simulink model "test_sim_non_linear_control_ver1"  (R2023a)
settings: Solver=FixedStepAuto  StartTime=0.0  StopTime=10.0  FixedStep=0.01  RelTol=1e-3
values from neighbouring files (symbols this model uses):
  e_init = y_init(2) - r_init(1)    [model_main_v10.m]
  K = Ke(:, 1:lenA)    [model_main_v10.m]
  KI = Ke(1, lenA+1:end)    [model_main_v10.m]
  x_init = [0 ... (first row only)    [model_main_v10.m]
libraries: simulink x2
settings Model: Creator=valer  LastModifiedBy=valer

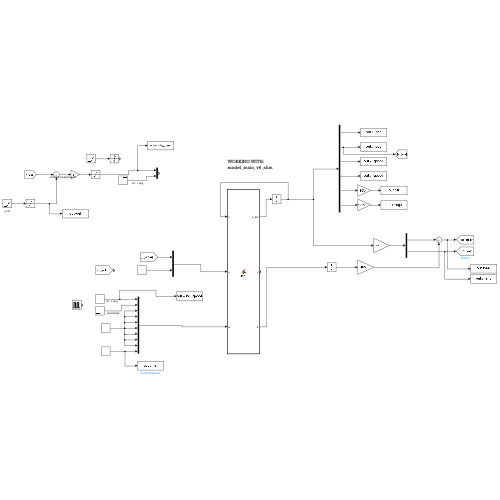
[thumbnail: Simulink's stored preview of the top-level diagram]
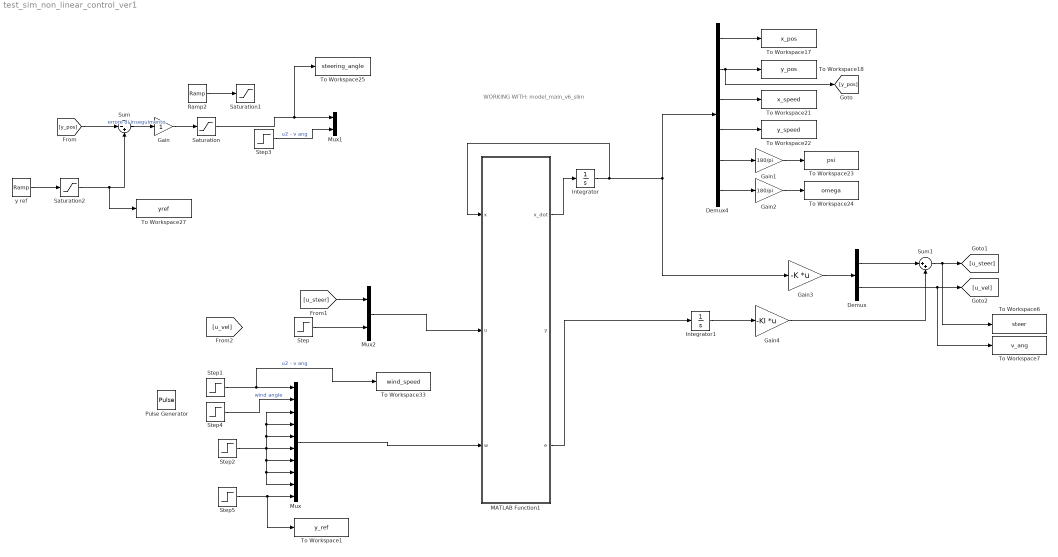
== system test_sim_non_linear_control_ver1 ==
  note: WORKING WITH:
      | model_main_v6_slim
  Demux : Demux  Outputs=2
  Demux4 : Demux  Outputs=6
  Gain : Gain
  Gain1 : Gain  Gain=180/pi
  Gain2 : Gain  Gain=180/pi
  Gain3 : Gain  Gain=-K  Multiplication=Matrix(K*u)
  Gain4 : Gain  Gain=-KI  Multiplication=Matrix(K*u)
  Integrator : Integrator  InitialCondition=x_init
  Integrator1 : Integrator  InitialCondition=e_init
  MATLAB Function1 : MATLAB Function  TreatAsAtomicUnit=on
  Mux : Mux  Inputs=10
  Mux1 : Mux  Inputs=2
  Mux2 : Mux  Inputs=2
  Pulse Generator : DiscretePulseGenerator  PulseType=Time based  Amplitude=0  Period=20  PulseWidth=50  PhaseDelay=1
  Ramp2 : simulink/Sources/Ramp  slope=0  start=1  InitialOutput=0
  Saturation : Saturate  UpperLimit=pi/4  LowerLimit=-pi/4
  Saturation1 : Saturate  UpperLimit=pi/36  LowerLimit=-pi/36
  Saturation2 : Saturate  UpperLimit=2.5  LowerLimit=-2.5
  Step : Step  Time=0  After=200  SampleTime=0
  Step1 : Step  After=0  SampleTime=0
  Step2 : Step  Time=0  Before=1  After=0  SampleTime=0
  Step3 : Step  Time=0  After=100  SampleTime=0
  Step4 : Step  After=0  SampleTime=0
  Step5 : Step  Time=0  Before=1  After=0  SampleTime=0
  Sum : Sum  Inputs=|-+
  Sum1 : Sum  Inputs=|++
  To Workspace1 : ToWorkspace  VariableName=y_ref  SaveFormat=Timeseries  SampleTime=-1
  To Workspace17 : ToWorkspace  VariableName=x_pos  SaveFormat=Timeseries  SampleTime=-1
  To Workspace18 : ToWorkspace  VariableName=y_pos  SaveFormat=Timeseries  SampleTime=-1
  To Workspace21 : ToWorkspace  VariableName=x_speed  SaveFormat=Timeseries  SampleTime=-1
  To Workspace22 : ToWorkspace  VariableName=y_speed  SaveFormat=Timeseries  SampleTime=-1
  To Workspace23 : ToWorkspace  VariableName=psi  SaveFormat=Timeseries  SampleTime=-1
  To Workspace24 : ToWorkspace  VariableName=omega  SaveFormat=Timeseries  SampleTime=-1
  To Workspace25 : ToWorkspace  VariableName=steering_angle  SaveFormat=Timeseries  SampleTime=-1
  To Workspace27 : ToWorkspace  VariableName=yref  SaveFormat=Timeseries  SampleTime=-1
  To Workspace33 : ToWorkspace  VariableName=wind_speed  SaveFormat=Timeseries  SampleTime=-1
  To Workspace6 : ToWorkspace  VariableName=steer  SaveFormat=Timeseries  SampleTime=-1
  To Workspace7 : ToWorkspace  VariableName=v_ang  SaveFormat=Timeseries  SampleTime=-1
  y ref : simulink/Sources/Ramp  slope=0  start=1  InitialOutput=0
  wires:
  Mux/1 -> MATLAB Function1/3(w)
  MATLAB Function1/1(x_dot) -> Integrator/1
  Integrator/1 -> MATLAB Function1/1(x), Gain3/1, Demux4/1
  Demux4/3 -> To Workspace21/1
  Demux4/1 -> To Workspace17/1
  Demux4/2 -> To Workspace18/1, [y_pos]
  Demux4/4 -> To Workspace22/1
  Step3/1 -> Mux1/2  "u2 - v ang"
  Step2/1 -> Mux/5, Mux/4, Mux/3, Mux/7, Mux/8, Mux/9, Mux/6
  Step4/1 -> Mux/2  "wind angle"
  [y_pos] -> Sum/1
  Sum/1 -> Gain/1  "errore di inseguimento"
  Gain/1 -> Saturation/1
  y ref/1 -> Saturation2/1
  Saturation2/1 -> To Workspace27/1, Sum/2
  Demux4/5 -> Gain1/1
  Gain2/1 -> To Workspace24/1
  Gain1/1 -> To Workspace23/1
  Demux4/6 -> Gain2/1
  Ramp2/1 -> Saturation1/1
  Step1/1 -> To Workspace33/1, Mux/1  "u2 - v ang"
  Saturation/1 -> To Workspace25/1, Mux1/1
  Sum1/1 -> [u_steer], To Workspace6/1
  Gain4/1 -> Sum1/2
  Demux/1 -> Sum1/1
  Demux/2 -> To Workspace7/1, [u_vel]
  Gain3/1 -> Demux/1
  Integrator1/1 -> Gain4/1
  MATLAB Function1/3(e) -> Integrator1/1
  Mux2/1 -> MATLAB Function1/2(u)
  [u_steer] -> Mux2/1
  Step/1 -> Mux2/2
  Step5/1 -> To Workspace1/1, Mux/10

== matlab function test_sim_non_linear_control_ver1/MATLAB Function1 ==
  data: x input; x_dot output; u input; y output; w input; e output


function [x_dot,y,e]= fcn(x, u, w)


% plant params for bus case
C1 = 1.2801; % [-] -> road fricition coefficients
C2 = 23.990;
C3 = 0.5200;
Cf = 1; % [-] -> aerodynamic drag coefficient front
Cs = 1.35; % [-] -> aerodynamic drag coefficient side
Sx = 7.5; % [m^2] -> longitunal projection area of the bus
Sy = 36; % [m^2] -> lateral projection area of the bus
g = 9.81; % [m/s^2] -> acceleration of gravity
lx = 5; % [m] -> distance from cg to wheel x coord
ly = 1.25; % [m] -> distance from cg to wheel y coord
mass = 22240; % [kg] -> mass of the bus
rho = 1.225; % [kg/m^3] -> air density
weight_part = 0.5; % [-] -> bus weight partition
epsilon = 1e-8; % [-] -> non 0/0 coeff
wheel_rad = 0.25; % [m] -> radius bus wheel


% plant formulas

Rbi = [cos(x(5)) sin(x(5)) 0;     % inertial-body
       -sin(x(5)) cos(x(5)) 0;
       0 0 1];

Rwb1 = [cos(u(1)) sin(u(1)) 0;  % body-wheel front wheels
       -sin(u(1)) cos(u(1)) 0;
       0 0 1];

Rwb3 = eye(3);  % wheel-body rear wheels
    

% calcolo dei mu

Pw1B = [lx ; ly ; 0];      % position vector of wheel i
Pw2B = [lx ; -ly ; 0];
Pw3B = [-lx ; -ly ; 0];
Pw4B = [-lx ; ly ; 0];
Pw1_2B = [lx; 0; 0];      % bycicle model positions
Pw3_4B = [-lx; 0; 0];

Rbi_der = [-sin(x(5)) cos(x(5)) 0;    % first derivative of Rbi
           -cos(x(5)) -sin(x(5)) 0;
           0 0 0];

VbI = [x(3); x(4); 0];  % intertial body velocity

Vw1I = VbI + Rbi_der' * Pw1_2B * x(6); % wheel speed in intertial
Vw3I = VbI + Rbi_der' * Pw3_4B * x(6);

Vw1W1 = Rwb1 * Rbi * Vw1I;    % wheel x speed in wheel
Vw3W3 = Rwb3 * Rbi * Vw3I;

% differenziale elettronico
delta_omega = sign(x(5)) * x(6) * ly/wheel_rad;

lambda1 = (u(2) * wheel_rad - Vw1W1(1)) / (epsilon + max(abs(u(2) * wheel_rad), abs(Vw1W1(1) ) ) );  % problem with max function
%beta1 = acos(Vw1W1(1)/sqrt(Vw1W1(1)^2 + Vw1W1(2)^2));
modulo1 = sqrt(Vw1W1(1)^2 + Vw1W1(2)^2);
beta1 = asin(Vw1W1(2)/modulo1);
mux1 = sign(lambda1) * C1 * (1 - exp(-C2 * abs(lambda1))) - C3 * lambda1;
muy1 = sign(-beta1/(pi/2)) * C1 * (1 - exp(-C2 * abs(-beta1/(pi/2)))) - C3 * (-beta1/(pi/2));

mux2 = mux1;
muy2 = muy1;

omega3 = u(2) + delta_omega;
lambda3 = (omega3 * wheel_rad - Vw3W3(1)) / (epsilon + max(abs(omega3 * wheel_rad), abs(Vw3W3(1))));
%beta3 = acos(Vw3W3(1)/sqrt(Vw3W3(1)^2 + Vw3W3(2)^2));
modulo3 = sqrt(Vw3W3(1)^2 + Vw3W3(2)^2);
beta3 = asin(Vw3W3(2)/modulo3);
mux3 = sign(lambda3) * C1 * (1 - exp(-C2 * abs(lambda3))) - C3 * lambda3;
muy3 = sign(-beta3/(pi/2)) * C1 * (1 - exp(-C2 * abs(-beta3/(pi/2)))) - C3 * (-beta3/(pi/2));

omega4 = u(2) - delta_omega;
lambda4 = (omega4 * wheel_rad - Vw3W3(1)) / (epsilon + max(abs(omega4 * wheel_rad), abs(Vw3W3(1))));
mux4 = sign(lambda4) * C1 * (1 - exp(-C2 * abs(lambda4))) - C3 * lambda4;
muy4 = muy3;

N1 = mass * g * weight_part * 0.5;
N2 = N1;

N3 = mass * g * (1 - weight_part) * 0.5;
N4 = N3;

Fw1xW1 = N1 * mux1;
Fw1yW1 = N1 * muy1;
Fw1W1 = [Fw1xW1; Fw1yW1; 0];

Fw2xW2 = N2 * mux2;
Fw2yW2 = N2 * muy2;
Fw2W2 = [Fw2xW2; Fw2yW2; 0];

Fw3xW3 = N3 * mux3;
Fw3yW3 = N3 * muy3;
Fw3W3 = [Fw3xW3; Fw3yW3; 0];

Fw4xW4 = N4 * mux4;   % wheel x forces
Fw4yW4 = N4 * muy4;   % wheel y forces
Fw4W4 = [Fw4xW4; Fw4yW4; 0];  % matrices of forces on each wheel

WxI = abs(w(1)) * cos(w(2));
%WxI = 0;
WyI = abs(w(1)) * sin(w(2));
WI = [WxI; WyI; 0];  % inertial wind speed

VaI = VbI + WI;  %WI;  % intertial total velocity

FaxI = 0.5 * rho * Sx * Cf * sign(VaI(1)) * norm(VaI(1))^2;  % aerodynamic x forces body
FayI = 0.5 * rho * Sy * Cs * sign(VaI(2)) * norm(VaI(2))^2;  % aerodynamic y forces body
FaI = [FaxI; FayI; 0];
FaB = Rbi * FaI;

%abI = (FaI + Rbi' * (Rwb1' *(Fw1W1) + Rwb1' *(Fw2W2) + Rwb3' *(Fw3W3) + Rwb3' *(Fw4W4)))/mass; % body acceleration in interial ref
FwB = Rwb1' *(Fw1W1) + Rwb1' *(Fw2W2) + Rwb3' *(Fw3W3) + Rwb3' *(Fw4W4);   % wheel forces in body coord
FwI = Rbi' * FwB;  % wheel forces in intertial coord
abI = (FaI + FwI)/mass;     % x and y total acc in intertial coord

% yaw moment

IzB = 275458;

laB = [lx; ly; 0];      % vector of body lenghts

MaB = cross(laB, FaB);%[0; 0; 0];%   % aerodynamic torque on body

Mw1B = cross(Pw1B, (Rwb1')*Fw1W1);   % torque on wheel i on body

Mw2B = cross(Pw2B, (Rwb1')*Fw2W2);

Mw3B = cross(Pw3B, (Rwb3')*Fw3W3);

Mw4B = cross(Pw4B, (Rwb3')*Fw4W4);

a_psi = (Mw1B + Mw2B + Mw3B + Mw4B + MaB)/ IzB;

% outputs

x_dot = [x(3);   % x speed
    x(4);        % y speed
    abI(1);      % x acceleration
    abI(2);      % y acceleration
    x(6);        % yaw rate
    a_psi(3)];   % yaw acceleration

y = [x(1) + w(3); % GPS x position
     x(2) + w(4); % visual system y position
     x(3) + w(5); % GPS x speed
     x(4) + w(6); % accelerometer/depth sensor y speed
     x(5) + w(7); % magnetic angular position sensor yaw angle
     x(6) + w(8)]; % gyroscope yaw rate


yaw_angle = x(5)*180/pi;

e = [x(2) - w(9); u(2) - w(10)];  % errors on references

MaBz = MaB(3);
Mw1Bz = Mw1B(3);
Mw2Bz = Mw2B(3);
Mw3Bz = Mw3B(3);
Mw4Bz = Mw4B(3);
acceleratore = 100;%FaB(1)/(N3+N4);
FaB = Rbi *FaI;
FaxB = FaB(1);
FayB = FaB(2);
FwxB = FwB(1);
FwyB = FwB(2);
lamb_max = max(abs(u(2) * wheel_rad), abs(Vw1W1(1)));
lamb_num = (u(2) * wheel_rad - Vw1W1(1));
Ftot = Rbi * abI;
Fxtot = Ftot(1);
Fwytot = Fw1yW1 + Fw2yW2 +Fw3yW3+ Fw4yW4;
Fytot = Ftot(2);
Mtot = a_psi(3);
Vtot = sqrt(VaI(1)^2 + VaI(2)^2);

%WIx = WxI;
